simulink model "ScriptDemo"  (R2022b)
settings: configuration reference "TmVcThermal_Configuration_sub" (kept outside this file)
undefined symbols (not defined in the file or in its folder): aaaa, bbbb, cTmComprCtrl_D_u8HvacFlowTable_db, cTmComprCtrl_D_u8HvacFlowTable_sw, cTmComprCtrl_n_i16ChillCmpIMax, cTmComprCtrl_n_i16ChillCmpIMin, cTmComprCtrl_n_i16ChillCmpIMin666, cTmComprCtrl_n_i16ChillCmpPMax, cTmComprCtrl_n_i16ChillCmpPMin, cTmComprCtrl_n_i16CmpChillCoolRpmKiMax, cTmComprCtrl_n_i16CmpChillCoolRpmKiMin, cTmComprCtrl_n_i16CmpChillCoolRpmKpMax, cTmComprCtrl_n_i16CmpChillCoolRpmKpMin, cTmComprCtrl_n_i16CmpCoolRpmKiMax, cTmComprCtrl_n_i16CmpCoolRpmKiMin, cTmComprCtrl_n_i16CmpCoolRpmKpMax, cTmComprCtrl_n_i16CmpCoolRpmKpMin, cTmComprCtrl_n_i16SM4CmpHeatKiMax, cTmComprCtrl_n_i16SM4CmpHeatKiMin, cTmComprCtrl_n_i16SM4CmpHeatKpMax, cTmComprCtrl_n_i16SM4CmpHeatKpMin, cTmComprCtrl_n_i16SM5CmpHeatKiMax, cTmComprCtrl_n_i16SM5CmpHeatKiMin, cTmComprCtrl_n_i16SM5CmpHeatKpMax, cTmComprCtrl_n_i16SM5CmpHeatKpMin, cTmComprCtrl_n_i16SM6CmpHeatKiMax, cTmComprCtrl_n_i16SM6CmpHeatKiMin, cTmComprCtrl_n_i16SM6CmpHeatKpMax, cTmComprCtrl_n_i16SM6CmpHeatKpMin, cTmComprCtrl_n_u16CmpMaxSpdFanFltLimt, cTmComprCtrl_n_u16CmpMaxSpdLoSidePFltLimt, cTmComprCtrl_n_u16CmpMaxSpdSensorFltLimt, cTmComprCtrl_n_u16CompMinRpm, cTmComprCtrl_n_u16CompRpmIncThres, cTmComprCtrl_t_u16BattCooltFFPeriod, cTmComprCtrl_t_u16BattCooltPIPeriod, cTmComprCtrl_t_u16CmpCoolFFPeriod, cTmComprCtrl_t_u16CmpCoolPIPeriod, cTmComprCtrl_t_u16CoolCmpChillFFPeriod, cTmComprCtrl_t_u16CoolCmpChillPIPeriod, cTmComprCtrl_t_u16SM4CmpHeatFFPeriod, cTmComprCtrl_t_u16SM4CmpHeatPIPeriod, cTmComprCtrl_t_u16SM5CmpHeatFFPeriod, cTmComprCtrl_t_u16SM5CmpHeatPIPeriod, cTmComprCtrl_t_u16SM6CmpHeatFFPeriod, cTmComprCtrl_t_u16SM6CmpHeatPIPeriod, cTmComprCtrl_Te_EvapClearInteg, cTmComprCtrl_Te_i16HpReqTempSaturoffset, cTmComprCtrl_Te_i16SatLpReplaceDiff, cTmComprCtrl_Te_i16SM3BatDiffStartEvapDecOffset, cTmComprCtrl_Te_i16SM3EvapLo, cTmComprCtrl_Te_i16SM3TBatDiffEntEvapDecOffset, cTmComprCtrl_Te_i16SM3TBatDiffEntEvapDecOffsetQuit, cTmComprCtrl_Te_s32ErrCmpChillPIContinueCoolH, cTmComprCtrl_Te_s32ErrCmpChillPIContinueCoolL, cTmComprCtrl_Te_s32ErrCmpPIContinueChillH, cTmComprCtrl_Te_s32ErrCmpPIContinueChillL, cTmComprCtrl_Te_s32ErrCmpPIContinueCoolH, cTmComprCtrl_Te_s32ErrCmpPIContinueCoolL, cTmComprCtrl_Te_s32ErrCmpPIContinueHeatH ... (+398)
libraries: simulink x846, PCMULib x711, simulink_need_slupdate x4
(part 13 of 49)

== system ScriptDemo/Find/findModBkSpecific/Before ==
  note: % 目的: 为输出端口创建debug 及对应的输入模块
      | [cnt] = createDebug(gcs)
  sTmRefriVlvCtrl_X_s32CEXVPosReqIn : Inport  OutDataTypeStr=single
  sTmRefriVlvCtrl_X_s32EEXVPosReqIn : Inport  Port=2  OutDataTypeStr=single
  sTmRefriVlvCtrl_X_s32BEXVPosReqIn : Inport  Port=3  OutDataTypeStr=single
  yTmRefriVlvCtrl_B_HpcCexvMovEnableIn : Inport  Port=4  OutDataTypeStr=boolean
  sTmRefriVlvCtrl_Z_u8CEXVInitStateIn : Inport  Port=5  OutDataTypeStr=uint8
  yTmRefriVlvCtrl_B_CexvCalibReqIn : Inport  Port=6  OutDataTypeStr=boolean
  yTmRefriVlvCtrl_B_HpcEexvMovEnableIn : Inport  Port=7  OutDataTypeStr=boolean
  sTmRefriVlvCtrl_Z_u8EEXVInitStateIn : Inport  Port=8  OutDataTypeStr=uint8
  yTmRefriVlvCtrl_B_EexvCalibReqIn : Inport  Port=9  OutDataTypeStr=boolean
  yTmRefriVlvCtrl_B_HpcBexvMovEnableIn : Inport  Port=10  OutDataTypeStr=boolean
  sTmRefriVlvCtrl_Z_u8BEXVInitStateIn : Inport  Port=11  OutDataTypeStr=uint8
  yTmRefriVlvCtrl_B_BexvCalibReqIn : Inport  Port=12  OutDataTypeStr=boolean
  sTmRefriVlvCtrl_X_s32SM3BexvMaxPosIn : Inport  Port=13  OutDataTypeStr=single
  yTmRefriVlvCtrl_B_EvapBattTLimBexvEnaIn : Inport  Port=14  OutDataTypeStr=boolean
  sTmRefriVlvCtrl_D_u8EexvRefriSwitchStIn : Inport  Port=15  OutDataTypeStr=uint8
  sTmRefriVlvCtrl_D_u8CexvRefriSwitchStIn : Inport  Port=16  OutDataTypeStr=uint8
  sTmRefriVlvCtrl_D_u8BexvRefriSwitchStIn : Inport  Port=17  OutDataTypeStr=uint8
  OutDebug : PCMULib/Interface/OutdebugRvs  SWI=cTmRefriVlvCtrl_X_s32CEXVPosReq_sw  DBI=cTmRefriVlvCtrl_X_s32CEXVPosReq_db
      settings: SourceProductName=PCMULib
  OutDebug1 : PCMULib/Interface/OutdebugRvs  SWI=cTmRefriVlvCtrl_X_s32EEXVPosReq_sw  DBI=cTmRefriVlvCtrl_X_s32EEXVPosReq_db
      settings: SourceProductName=PCMULib
  OutDebug10 : PCMULib/Interface/OutdebugRvs  SWI=cTmRefriVlvCtrl_Z_u8BEXVInitState_sw  DBI=cTmRefriVlvCtrl_Z_u8BEXVInitState_db
      settings: SourceProductName=PCMULib
  OutDebug11 : PCMULib/Interface/OutdebugRvs  SWI=cTmRefriVlvCtrl_B_BexvCalibReq_sw  DBI=cTmRefriVlvCtrl_B_BexvCalibReq_db
      settings: SourceProductName=PCMULib
  OutDebug12 : PCMULib/Interface/OutdebugRvs  SWI=cTmRefriVlvCtrl_X_s32SM3BexvMaxPos_sw  DBI=cTmRefriVlvCtrl_X_s32SM3BexvMaxPos_db
      settings: SourceProductName=PCMULib
  OutDebug13 : PCMULib/Interface/OutdebugRvs  SWI=cTmRefriVlvCtrl_B_EvapBattTLimBexvEna_sw  DBI=cTmRefriVlvCtrl_B_EvapBattTLimBexvEna_db
      settings: SourceProductName=PCMULib
  OutDebug14 : PCMULib/Interface/OutdebugRvs  SWI=cTmRefriVlvCtrl_D_u8EexvRefriSwitchSt_sw  DBI=cTmRefriVlvCtrl_D_u8EexvRefriSwitchSt_db
      settings: SourceProductName=PCMULib
  OutDebug15 : PCMULib/Interface/OutdebugRvs  SWI=cTmRefriVlvCtrl_D_u8CexvRefriSwitchSt_sw  DBI=cTmRefriVlvCtrl_D_u8CexvRefriSwitchSt_db
      settings: SourceProductName=PCMULib
  OutDebug16 : PCMULib/Interface/OutdebugRvs  SWI=cTmRefriVlvCtrl_D_u8BexvRefriSwitchSt_sw  DBI=cTmRefriVlvCtrl_D_u8BexvRefriSwitchSt_db
      settings: SourceProductName=PCMULib
  OutDebug2 : PCMULib/Interface/OutdebugRvs  SWI=cTmRefriVlvCtrl_X_s32BEXVPosReq_sw  DBI=cTmRefriVlvCtrl_X_s32BEXVPosReq_db
      settings: SourceProductName=PCMULib
  OutDebug3 : PCMULib/Interface/OutdebugRvs  SWI=cTmRefriVlvCtrl_B_HpcCexvMovEnable_sw  DBI=cTmRefriVlvCtrl_B_HpcCexvMovEnable_db
      settings: SourceProductName=PCMULib
  OutDebug4 : PCMULib/Interface/OutdebugRvs  SWI=cTmRefriVlvCtrl_Z_u8CEXVInitState_sw  DBI=cTmRefriVlvCtrl_Z_u8CEXVInitState_db
      settings: SourceProductName=PCMULib
  OutDebug5 : PCMULib/Interface/OutdebugRvs  SWI=cTmRefriVlvCtrl_B_CexvCalibReq_sw  DBI=cTmRefriVlvCtrl_B_CexvCalibReq_db
      settings: SourceProductName=PCMULib
  OutDebug6 : PCMULib/Interface/OutdebugRvs  SWI=cTmRefriVlvCtrl_B_HpcEexvMovEnable_sw  DBI=cTmRefriVlvCtrl_B_HpcEexvMovEnable_db
      settings: SourceProductName=PCMULib
  OutDebug7 : PCMULib/Interface/OutdebugRvs  SWI=cTmRefriVlvCtrl_Z_u8EEXVInitState_sw  DBI=cTmRefriVlvCtrl_Z_u8EEXVInitState_db
      settings: SourceProductName=PCMULib
  OutDebug8 : PCMULib/Interface/OutdebugRvs  SWI=cTmRefriVlvCtrl_B_EexvCalibReq_sw  DBI=cTmRefriVlvCtrl_B_EexvCalibReq_db
      settings: SourceProductName=PCMULib
  OutDebug9 : PCMULib/Interface/OutdebugRvs  SWI=cTmRefriVlvCtrl_B_HpcBexvMovEnable_sw  DBI=cTmRefriVlvCtrl_B_HpcBexvMovEnable_db
      settings: SourceProductName=PCMULib
  sTmRefriVlvCtrl_X_s32CEXVPosReq : Outport  OutDataTypeStr=single
  sTmRefriVlvCtrl_X_s32EEXVPosReq : Outport  Port=2  OutDataTypeStr=single
  sTmRefriVlvCtrl_X_s32BEXVPosReq : Outport  Port=3  OutDataTypeStr=single
  yTmRefriVlvCtrl_B_HpcCexvMovEnable : Outport  Port=4  OutDataTypeStr=boolean
  sTmRefriVlvCtrl_Z_u8CEXVInitState : Outport  Port=5  OutDataTypeStr=uint8
  yTmRefriVlvCtrl_B_CexvCalibReq : Outport  Port=6  OutDataTypeStr=boolean
  yTmRefriVlvCtrl_B_HpcEexvMovEnable : Outport  Port=7  OutDataTypeStr=boolean
  sTmRefriVlvCtrl_Z_u8EEXVInitState : Outport  Port=8  OutDataTypeStr=uint8
  yTmRefriVlvCtrl_B_EexvCalibReq : Outport  Port=9  OutDataTypeStr=boolean
  yTmRefriVlvCtrl_B_HpcBexvMovEnable : Outport  Port=10  OutDataTypeStr=boolean
  sTmRefriVlvCtrl_Z_u8BEXVInitState : Outport  Port=11  OutDataTypeStr=uint8
  yTmRefriVlvCtrl_B_BexvCalibReq : Outport  Port=12  OutDataTypeStr=boolean
  sTmRefriVlvCtrl_X_s32SM3BexvMaxPos : Outport  Port=13  OutDataTypeStr=single
  yTmRefriVlvCtrl_B_EvapBattTLimBexvEna : Outport  Port=14  OutDataTypeStr=boolean
  sTmRefriVlvCtrl_D_u8EexvRefriSwitchSt : Outport  Port=15  OutDataTypeStr=uint8
  sTmRefriVlvCtrl_D_u8CexvRefriSwitchSt : Outport  Port=16  OutDataTypeStr=uint8
  sTmRefriVlvCtrl_D_u8BexvRefriSwitchSt : Outport  Port=17  OutDataTypeStr=uint8
  wires:
  sTmRefriVlvCtrl_X_s32SM3BexvMaxPosIn/1 -> OutDebug12/1
  OutDebug12/1 -> sTmRefriVlvCtrl_X_s32SM3BexvMaxPos/1
  sTmRefriVlvCtrl_X_s32BEXVPosReqIn/1 -> OutDebug2/1
  OutDebug2/1 -> sTmRefriVlvCtrl_X_s32BEXVPosReq/1
  OutDebug16/1 -> sTmRefriVlvCtrl_D_u8BexvRefriSwitchSt/1
  sTmRefriVlvCtrl_D_u8EexvRefriSwitchStIn/1 -> OutDebug14/1
  OutDebug5/1 -> yTmRefriVlvCtrl_B_CexvCalibReq/1
  OutDebug3/1 -> yTmRefriVlvCtrl_B_HpcCexvMovEnable/1
  sTmRefriVlvCtrl_Z_u8CEXVInitStateIn/1 -> OutDebug4/1
  OutDebug4/1 -> sTmRefriVlvCtrl_Z_u8CEXVInitState/1
  sTmRefriVlvCtrl_D_u8BexvRefriSwitchStIn/1 -> OutDebug16/1
  OutDebug1/1 -> sTmRefriVlvCtrl_X_s32EEXVPosReq/1
  OutDebug14/1 -> sTmRefriVlvCtrl_D_u8EexvRefriSwitchSt/1
  yTmRefriVlvCtrl_B_CexvCalibReqIn/1 -> OutDebug5/1
  sTmRefriVlvCtrl_X_s32EEXVPosReqIn/1 -> OutDebug1/1
  yTmRefriVlvCtrl_B_HpcCexvMovEnableIn/1 -> OutDebug3/1
  yTmRefriVlvCtrl_B_EvapBattTLimBexvEnaIn/1 -> OutDebug13/1
  OutDebug13/1 -> yTmRefriVlvCtrl_B_EvapBattTLimBexvEna/1
  sTmRefriVlvCtrl_Z_u8BEXVInitStateIn/1 -> OutDebug10/1
  OutDebug10/1 -> sTmRefriVlvCtrl_Z_u8BEXVInitState/1
  sTmRefriVlvCtrl_D_u8CexvRefriSwitchStIn/1 -> OutDebug15/1
  OutDebug15/1 -> sTmRefriVlvCtrl_D_u8CexvRefriSwitchSt/1
  OutDebug/1 -> sTmRefriVlvCtrl_X_s32CEXVPosReq/1
  OutDebug7/1 -> sTmRefriVlvCtrl_Z_u8EEXVInitState/1
  OutDebug8/1 -> yTmRefriVlvCtrl_B_EexvCalibReq/1
  yTmRefriVlvCtrl_B_EexvCalibReqIn/1 -> OutDebug8/1
  sTmRefriVlvCtrl_X_s32CEXVPosReqIn/1 -> OutDebug/1
  OutDebug6/1 -> yTmRefriVlvCtrl_B_HpcEexvMovEnable/1
  yTmRefriVlvCtrl_B_HpcEexvMovEnableIn/1 -> OutDebug6/1
  sTmRefriVlvCtrl_Z_u8EEXVInitStateIn/1 -> OutDebug7/1
  yTmRefriVlvCtrl_B_HpcBexvMovEnableIn/1 -> OutDebug9/1
  OutDebug9/1 -> yTmRefriVlvCtrl_B_HpcBexvMovEnable/1
  yTmRefriVlvCtrl_B_BexvCalibReqIn/1 -> OutDebug11/1
  OutDebug11/1 -> yTmRefriVlvCtrl_B_BexvCalibReq/1

== system ScriptDemo/Find/findNameMdOut/SM1 ==
  In : Inport
  rSM1_D_u32AccmKp : Outport
  wires:
  In/1 -> rSM1_D_u32AccmKp/1

== system ScriptDemo/Find/findNameMdOut/SM2 ==
  In : Inport
  rSM2_D_u32AccmKp : Outport
  wires:
  In/1 -> rSM2_D_u32AccmKp/1

== system ScriptDemo/Find/findNameMdOut/SM3 ==
  In : Inport
  sTmComprCtrl_D_u32AccmKpSM3 : Outport
  wires:
  In/1 -> sTmComprCtrl_D_u32AccmKpSM3/1

== system ScriptDemo/Find/findNameMdOut/SM4 ==
  In : Inport
  sTmComprCtrl_D_u32AccmKpSM4 : Outport
  wires:
  In/1 -> sTmComprCtrl_D_u32AccmKpSM4/1

== system ScriptDemo/WorkFlow/Step1_CreateSoftwareReq/Fun666666_Req26245_DemoSub1 ==
  note: 压缩机不满足开启条件
  note: 压缩机允许功率
  note: 压缩机满足开启条件
  note: <模型信息: Fun666666_Req26245_DemoSub1>
      |
      | 【输入端口】
      | sTmIn_Pw_s32HvCoolgAllwd
      | xTmComprCtrl_B_CompOnReqCompOn
      |
      | 【输出端口】
      | sTmComprCtrl_Pw_s32ElacCmprMaxState
      | yTmComprCtrl_B_HpcCoolgLimd
      |
      | 【标定量】
      | cTmComprCtrl_n_i16ChillCmpIMin
      |
      | 创建时间: 2025-03-13 10:25:04
  sTmIn_Pw_s32HvCoolgAllwd : Inport  OutDataTypeStr=single
  xTmComprCtrl_B_CompOnReqCompOn : Inport  Port=2  OutDataTypeStr=boolean
  Compare To Constant : simulink/Logic and Bit Operations/Compare To Constant  relop=>=  const=6500  OutDataTypeStr=boolean
  Compare To Constant1 : simulink/Logic and Bit Operations/Compare To Constant  relop===  const=6500  OutDataTypeStr=boolean
  Constant1 : Constant  Commented=on  Value=cTmComprCtrl_n_i16ChillCmpIMin666  OutDataTypeStr=single
  Constant2 : Constant  Value=cTmComprCtrl_n_i16ChillCmpIMin  OutDataTypeStr=single
  Constant4 : Constant  Value=6500  OutDataTypeStr=single
  Relay : Relay  Commented=on  OnSwitchValue=aaaa  OffSwitchValue=bbbb
  Switch1 : Switch  Criteria=u2 ~= 0  SaturateOnIntegerOverflow=off  InputSameDT=off
  Switch3 : Switch  Criteria=u2 ~= 0  Threshold=6500  SaturateOnIntegerOverflow=off  InputSameDT=off
  sTmComprCtrl_Pw_s32ElacCmprMaxState : Outport  OutDataTypeStr=single
  yTmComprCtrl_B_HpcCoolgLimd : Outport  Port=2  OutDataTypeStr=boolean
  wires:
  Compare To Constant1/1 -> [yTmComprCtrl_B_HpcCoolgLimd]
  Switch1/1 -> [sTmComprCtrl_Pw_s32ElacCmprMaxState], Compare To Constant1/1
  Constant2/1 -> Switch1/3
  Constant4/1 -> Switch3/1
  Compare To Constant/1 -> Switch3/2
  Switch3/1 -> Switch1/1
  [xTmComprCtrl_B_CompOnReqCompOn] -> Switch1/2
  [sTmIn_Pw_s32HvCoolgAllwd] -> Switch3/3, Compare To Constant/1
  sTmIn_Pw_s32HvCoolgAllwd/1 -> [sTmIn_Pw_s32HvCoolgAllwd]
  xTmComprCtrl_B_CompOnReqCompOn/1 -> [xTmComprCtrl_B_CompOnReqCompOn]
  [sTmComprCtrl_Pw_s32ElacCmprMaxState] -> sTmComprCtrl_Pw_s32ElacCmprMaxState/1
  [yTmComprCtrl_B_HpcCoolgLimd] -> yTmComprCtrl_B_HpcCoolgLimd/1

== system ScriptDemo/WorkFlow/Step1_CreateSoftwareReq/Fun666666_Req26246_DemoSub2 ==

== system ScriptDemo/WorkFlow/Step1_CreateSoftwareReq/Fun666666_Req26247_DemoSub3 ==

== system ScriptDemo/WorkFlow/Step1_CreateSoftwareReq/Fun666666_Req26248_DemoSub4 ==

== system ScriptDemo/WorkFlow/Step1_CreateSoftwareReq/Fun666666_Req26249_DemoSub5 ==

== system ScriptDemo/WorkFlow/Step1_CreateSoftwareReq/Fun888888_Req26250_DemoSub6 ==

== system ScriptDemo/WorkFlow/Step1_CreateSoftwareReq/Fun888888_Req26251_DemoSub7 ==

== system ScriptDemo/WorkFlow/Step1_CreateSoftwareReq/Fun888888_Req26252_DemoSub8 ==

== system ScriptDemo/WorkFlow/Step1_CreateSoftwareReq/Fun888888_Req26253_DemoSub9 ==

== system ScriptDemo/WorkFlow/Step1_CreateSoftwareReq/Fun888888_Req26254_DemoSub10 ==

== system ScriptDemo/WorkFlow/Step1_CreateSubModel/Fun666666_Req26245_DemoSub1 ==

== system ScriptDemo/WorkFlow/Step1_CreateSubModel/Fun666666_Req26246_DemoSub2 ==

== system ScriptDemo/WorkFlow/Step1_CreateSubModel/Fun666666_Req26247_DemoSub3 ==

== system ScriptDemo/WorkFlow/Step1_CreateSubModel/Fun666666_Req26248_DemoSub4 ==

== system ScriptDemo/WorkFlow/Step1_CreateSubModel/Fun666666_Req26249_DemoSub5 ==

== system ScriptDemo/WorkFlow/Step1_CreateSubModel/Fun888888_Req26250_DemoSub6 ==

== system ScriptDemo/WorkFlow/Step1_CreateSubModel/Fun888888_Req26251_DemoSub7 ==

== system ScriptDemo/WorkFlow/Step1_CreateSubModel/Fun888888_Req26252_DemoSub8 ==

== system ScriptDemo/WorkFlow/Step1_CreateSubModel/Fun888888_Req26253_DemoSub9 ==

== system ScriptDemo/WorkFlow/Step1_CreateSubModel/Fun888888_Req26254_DemoSub10 ==

== system ScriptDemo/createHarness/ID31659_OffCodeState/bk ==
  note: 第1位
  note: 输出: 0
  note: 输出: 4
  note: 第5位
  note: 第24位
  note: 第5、6、10、13、25、26位
  note: 第8位
  note: 输出: 1
  note: 输出: 5
  note: 输出: 3
  note: 输出: 2
  note: 第3、4、7、15、16、17、18、19、20、21、22、23、27、28、29、30
  note: 输出: 6
  note: 输出: 7
  sTmComprCtrl_D_u32AcOffCode : Inport  OutDataTypeStr=uint32
  sTmRefriModeMgr_D_u8HPCurMode : Inport  Port=2
  Bitwise Operator : simulink/Logic and Bit Operations/Bitwise Operator  logicop=AND  UseBitMask=on  BitMask=0x00000001  BitMaskRealWorld=Stored Integer
  Bitwise Operator2 : simulink/Logic and Bit Operations/Bitwise Operator  logicop=AND  UseBitMask=on  BitMask=0x01000000  BitMaskRealWorld=Stored Integer
  Bitwise Operator3 : simulink/Logic and Bit Operations/Bitwise Operator  logicop=AND  UseBitMask=on  BitMask=0x00000100  BitMaskRealWorld=Stored Integer
  Bitwise Operator4 : simulink/Logic and Bit Operations/Bitwise Operator  logicop=AND  UseBitMask=on  BitMask=0x20  BitMaskRealWorld=Stored Integer
  Bitwise Operator5 : simulink/Logic and Bit Operations/Bitwise Operator  logicop=AND  UseBitMask=on  BitMask=0x78FF804C  BitMaskRealWorld=Stored Integer
  Bitwise Operator6 : simulink/Logic and Bit Operations/Bitwise Operator  logicop=AND  UseBitMask=on  BitMask=0x06002460  BitMaskRealWorld=Stored Integer
  Compare To Constant{,1..7} (8 alike) : simulink/Logic and Bit Operations/Compare To Constant  relop=>  const=0  OutDataTypeStr=uint8
  Constant : Constant  Value=0  OutDataTypeStr=uint64
  Constant1 : Constant  Value=[1 21 3 23]  OutDataTypeStr=uint64
  Constant2 : Constant  Value=[2 22 4 5 6 7]  OutDataTypeStr=uint64
  Logical Operator : Logic  AllPortsSameDT=off  OutDataTypeStr=boolean
  Logical Operator1 : Logic  Operator=OR  Inputs=1  AllPortsSameDT=off  OutDataTypeStr=boolean
  Logical Operator2 : Logic  Operator=OR  Inputs=1  AllPortsSameDT=off  OutDataTypeStr=boolean
  Logical Operator3 : Logic  AllPortsSameDT=off  OutDataTypeStr=boolean
  Merge : Merge  Inputs=8
  Relational Operator : RelationalOperator  Operator===  OutDataTypeStr=boolean  RndMeth=Simplest  InputSameDT=off
  Relational Operator1 : RelationalOperator  Operator===  OutDataTypeStr=boolean  RndMeth=Simplest  InputSameDT=off
  Relational Operator2 : RelationalOperator  Operator===  OutDataTypeStr=boolean  RndMeth=Simplest  InputSameDT=off
  Subsystem : Subsystem
  Subsystem1 : Subsystem
  Subsystem2 : Subsystem
  Subsystem3 : Subsystem
  Subsystem4 : Subsystem
  Subsystem5 : Subsystem
  Subsystem6 : Subsystem
  Subsystem7 : Subsystem
  sTmComprCtrl_D_u8AirCondCmpsrStats : Outport  OutDataTypeStr=uint8
  wires:
  Compare To Constant2/1 -> Subsystem2/Enable
  sTmComprCtrl_D_u32AcOffCode/1 -> Relational Operator/1, Bitwise Operator6/1, Bitwise Operator5/1, Bitwise Operator4/1, Bitwise Operator3/1, Bitwise Operator2/1, Bitwise Operator/1
  Subsystem5/1(sTmComprCtrl_D_u8AirCondCmpsrStats) -> Merge/6
  Compare To Constant6/1 -> Subsystem6/Enable
  Constant2/1 -> Relational Operator2/2
  Subsystem7/1(sTmComprCtrl_D_u8AirCondCmpsrStats) -> Merge/8
  Logical Operator3/1 -> Compare To Constant7/1
  Subsystem/1(sTmComprCtrl_D_u8AirCondCmpsrStats) -> Merge/1
  Relational Operator/1 -> Logical Operator3/1, Logical Operator/1
  Compare To Constant4/1 -> Subsystem4/Enable
  Merge/1 -> sTmComprCtrl_D_u8AirCondCmpsrStats/1
  Constant1/1 -> Relational Operator1/2
  Bitwise Operator2/1 -> Compare To Constant1/1
  Subsystem6/1(sTmComprCtrl_D_u8AirCondCmpsrStats) -> Merge/7
  Subsystem2/1(sTmComprCtrl_D_u8AirCondCmpsrStats) -> Merge/3
  Subsystem1/1(sTmComprCtrl_D_u8AirCondCmpsrStats) -> Merge/2
  Bitwise Operator6/1 -> Compare To Constant5/1
  Relational Operator1/1 -> Logical Operator1/1
  Subsystem4/1(sTmComprCtrl_D_u8AirCondCmpsrStats) -> Merge/5
  Bitwise Operator5/1 -> Compare To Constant4/1
  Subsystem3/1(sTmComprCtrl_D_u8AirCondCmpsrStats) -> Merge/4
  Relational Operator2/1 -> Logical Operator2/1
  Logical Operator/1 -> Compare To Constant6/1
  Bitwise Operator/1 -> Compare To Constant/1
  Compare To Constant3/1 -> Subsystem3/Enable
  Bitwise Operator3/1 -> Compare To Constant2/1
  sTmRefriModeMgr_D_u8HPCurMode/1 -> Relational Operator2/1, Relational Operator1/1
  Compare To Constant/1 -> Subsystem/Enable
  Bitwise Operator4/1 -> Compare To Constant3/1
  Logical Operator1/1 -> Logical Operator/2
  Compare To Constant7/1 -> Subsystem7/Enable
  Compare To Constant1/1 -> Subsystem1/Enable
  Constant/1 -> Relational Operator/2
  Logical Operator2/1 -> Logical Operator3/2
  Compare To Constant5/1 -> Subsystem5/Enable

== system ScriptDemo/Change/changeModSize/After/Subsystem ==
  sTmSigProces_Te_s32EvapFanReqRamp : Inport  OutDataTypeStr=single
  sTmDiag_D_u8TeEvapFltSt : Inport  Port=2  OutDataTypeStr=uint8
  sTmIn_D_u8HeatPump : Inport  Port=3  OutDataTypeStr=uint8
  sTmIn_X_s32ClimtRcirc : Inport  Port=4  OutDataTypeStr=single
  sTmComprCtrl_D_u8HvacFlowLevel : Inport  Port=5  OutDataTypeStr=uint8
  sTmSigProces_Te_s32EvapFanFilter : Inport  Port=6  OutDataTypeStr=single
  sTmSigProces_Te_s32SatLp : Inport  Port=7  OutDataTypeStr=single
  xTmComprCtrl_B_CompOnReqCompOn : Inport  Port=8  OutDataTypeStr=boolean
  yTmRefriModeMgr_B_CoolOCRMode : Inport  Port=9  OutDataTypeStr=boolean
  sTmSigProces_Pw_i16ReqPwrForCool : Inport  Port=10  OutDataTypeStr=int16
  rSM2SM22_n_u16DisOverrideValue : Outport  OutDataTypeStr=uint16
  rSM2SM22_t_u16PIPeriod : Outport  Port=2  OutDataTypeStr=uint16
  rSM2SM22_Te_s32UpErrStop : Outport  Port=3  OutDataTypeStr=single
  rSM2SM22_n_u16ComprRpmFF : Outport  Port=4  OutDataTypeStr=uint16
  rSM2SM22_n_u16ComprRpmKp : Outport  Port=5  OutDataTypeStr=uint16
  rSM2SM22_n_u16ComprRpmKi : Outport  Port=6  OutDataTypeStr=uint16
  rSM2SM22_Te_s32LowErrStop : Outport  Port=7  OutDataTypeStr=single
  rSM2SM22_n_i16KpUpLimit : Outport  Port=8  OutDataTypeStr=int16
  rSM2SM22_n_i16KpLowLimit : Outport  Port=9  OutDataTypeStr=int16
  rSM2SM22_n_i16KiUpLimit : Outport  Port=10  OutDataTypeStr=int16
  rSM2SM22_n_i16KiLowLimit : Outport  Port=11  OutDataTypeStr=int16
  rSM2SM22_B_Enable : Outport  Port=12  OutDataTypeStr=boolean
  rSM2SM22_Te_s32TempError : Outport  Port=13  OutDataTypeStr=single
  wires:
  sTmSigProces_Te_s32SatLp/1 -> [sTmSigProces_Te_s32SatLp]
  [rTmComprCtrl_n_u16ComprRpmKp] -> rSM2SM22_n_u16ComprRpmKp/1
  sTmDiag_D_u8TeEvapFltSt/1 -> [sTmDiag_D_u8TeEvapFltSt]
  sTmIn_X_s32ClimtRcirc/1 -> [sTmIn_X_s32ClimtRcirc]
  sTmSigProces_Te_s32EvapFanReqRamp/1 -> [sTmSigProces_Te_s32EvapFanReqRamp]
  sTmIn_D_u8HeatPump/1 -> [sTmIn_D_u8HeatPump]
  sTmSigProces_Te_s32EvapFanFilter/1 -> [sTmSigProces_Te_s32EvapFanFilter]
  [rTmComprCtrl_n_u16ComprRpmFF] -> rSM2SM22_n_u16ComprRpmFF/1
  xTmComprCtrl_B_CompOnReqCompOn/1 -> [xTmComprCtrl_B_CompOnReqCompOn]
  [rTmComprCtrl_Te_s32UpErrStop] -> rSM2SM22_Te_s32UpErrStop/1
  [rTmComprCtrl_t_u16PIPeriod] -> rSM2SM22_t_u16PIPeriod/1
  ? -> [yTmRefriModeMgr_B_CoolModeInCycle]
  sTmComprCtrl_D_u8HvacFlowLevel/1 -> [sTmComprCtrl_D_u8HvacFlowLevel]
  ? -> [sTmSigProces_Te_s32TAmb]
  [rTmComprCtrl_Te_s32TempError] -> rSM2SM22_Te_s32TempError/1
  [rTmComprCtrl_n_i16KiUpLimit] -> rSM2SM22_n_i16KiUpLimit/1
  [rTmComprCtrl_Te_s32LowErrStop] -> rSM2SM22_Te_s32LowErrStop/1
  [rTmComprCtrl_n_i16KiLowLimit] -> rSM2SM22_n_i16KiLowLimit/1
  [rTmComprCtrl_n_i16KpLowLimit] -> rSM2SM22_n_i16KpLowLimit/1
  yTmRefriModeMgr_B_CoolOCRMode/1 -> [yTmRefriModeMgr_B_CoolOCRMode]
  [rTmComprCtrl_n_i16KpUpLimit] -> rSM2SM22_n_i16KpUpLimit/1
  sTmSigProces_Pw_i16ReqPwrForCool/1 -> [sTmSigProces_Pw_i16ReqPwrForCool]
  [xTmComprCtrl_B_Enable] -> rSM2SM22_B_Enable/1
  [rTmComprCtrl_n_u16DisOverrideValue] -> rSM2SM22_n_u16DisOverrideValue/1
  [rTmComprCtrl_n_u16ComprRpmKi] -> rSM2SM22_n_u16ComprRpmKi/1

== system ScriptDemo/Change/changeModSizeGcs/Before/Subsystem ==
  rTmComprCtrl_n_u16CompRpmReqModeOut : Inport  OutDataTypeStr=uint16
  sTmDiag_D_u8CmprDischrgTFltSt : Inport  Port=2  OutDataTypeStr=uint8
  sTmDiag_D_u8FanFltSt : Inport  Port=3  OutDataTypeStr=uint8
  sTmDiag_D_u8HiSidePFltSt : Inport  Port=4  OutDataTypeStr=uint8
  sTmDiag_D_u8OutrCondOutTFltSt : Inport  Port=5  OutDataTypeStr=uint8
  sTmIn_n_s32ElacCmprActl : Inport  Port=6  OutDataTypeStr=single
  sTmIn_v_s32VehSpdLgt : Inport  Port=7  OutDataTypeStr=single
  sTmRefriModeMgr_D_u8HpFmCmd : Inport  Port=8  OutDataTypeStr=uint8
  sTmSigProces_Pw_i16ReqPwrForHeat : Inport  Port=9  OutDataTypeStr=int16
  sTmSigProces_Te_s32CompDischarge : Inport  Port=10  OutDataTypeStr=single
  sTmSigProces_md_u16BlwCool : Inport  Port=11  OutDataTypeStr=uint16
  sTmSigProces_p_u16PHighSide : Inport  Port=12  OutDataTypeStr=uint16
  sTmSigProces_p_u16PLowSide : Inport  Port=13  OutDataTypeStr=uint16
  sTmIn_D_u8HeatPump : Inport  Port=14  OutDataTypeStr=uint8
  sTmIn_D_u8ElecDriveline : Inport  Port=15
  sTmSigProces_md_u16BlwHeat : Inport  Port=16  OutDataTypeStr=uint16
  sTmDiag_D_u8LoSidePFltSt : Inport  Port=17  OutDataTypeStr=uint8
  xTmComprCtrl_B_CompOnReqCompOn : Inport  Port=18  OutDataTypeStr=boolean
  rTmComprCtrl_n_u16CompRpmReqFilter : Outport  OutDataTypeStr=uint16
  xTmComprCtrl_B_KeepRpm : Outport  Port=2  OutDataTypeStr=boolean
  xFilter_B_ComprStop : Outport  Port=3  OutDataTypeStr=boolean
  sFilter_n_u16CompMaxRpm : Outport  Port=4  OutDataTypeStr=uint16
  rFilter_p_u16AcHiSideHiCut : Outport  Port=5  OutDataTypeStr=uint16
  rFilter_p_u16CmpLimitNormalP : Outport  Port=6  OutDataTypeStr=uint16
  rFilter_p_u16CmpLimitLowP : Outport  Port=7  OutDataTypeStr=uint16
  rFilter_p_u16CmpLimitMidP : Outport  Port=8  OutDataTypeStr=uint16
  rFilter_p_u16CmpLimitShutDownP : Outport  Port=9  OutDataTypeStr=uint16
  xTmComprCtrl_B_ReduceRpm : Outport  Port=10  OutDataTypeStr=boolean
  wires:
  ? -> [sTmRefriModeMgr_D_u8HPCurMode]
  sTmIn_n_s32ElacCmprActl/1 -> [sTmIn_n_s32ElacCmprActl]
  [rTmComprCtrl_p_u16AcHiSideHiCut] -> rFilter_p_u16AcHiSideHiCut/1
  sTmIn_D_u8HeatPump/1 -> [sTmIn_D_u8HeatPump]
  sTmSigProces_md_u16BlwCool/1 -> [sTmSigProces_md_u16BlwCool]
  sTmDiag_D_u8OutrCondOutTFltSt/1 -> [sTmDiag_D_u8OutrCondOutTFltSt]
  ? -> [sTmSigProces_Te_s32TAmb]
  sTmSigProces_md_u16BlwHeat/1 -> [sTmSigProces_md_u16BlwHeat]
  [rTmComprCtrl_p_u16CmpLimitShutDownP] -> rFilter_p_u16CmpLimitShutDownP/1
  sTmRefriModeMgr_D_u8HpFmCmd/1 -> [sTmRefriModeMgr_D_u8HpFmCmd]
  [rTmComprCtrl_p_u16CmpLimitLowP] -> rFilter_p_u16CmpLimitLowP/1
  sTmDiag_D_u8LoSidePFltSt/1 -> [sTmDiag_D_u8LoSidePFltSt]
  sTmSigProces_p_u16PLowSide/1 -> [sTmSigProces_p_u16PLowSide]
  [rTmComprCtrl_n_u16CompRpmReqCompOn] -> rTmComprCtrl_n_u16CompRpmReqFilter/1
  [xTmComprCtrl_B_ComprStop] -> xFilter_B_ComprStop/1
  sTmIn_D_u8ElecDriveline/1 -> [sTmIn_D_u8ElecDriveline]
  sTmDiag_D_u8HiSidePFltSt/1 -> [sTmDiag_D_u8HiSidePFltSt]
  [sTmComprCtrl_n_u16CompMaxRpm] -> sFilter_n_u16CompMaxRpm/1
  ? -> [sTmSigProces_D_u8CarChrgMode]
  [xTmComprCtrl_B_KeepRpm] -> xTmComprCtrl_B_KeepRpm/1
  sTmDiag_D_u8CmprDischrgTFltSt/1 -> [sTmDiag_D_u8CmprDischrgTFltSt]
  sTmSigProces_p_u16PHighSide/1 -> [sTmSigProces_p_u16PHighSide]
  xTmComprCtrl_B_CompOnReqCompOn/1 -> [xTmComprCtrl_B_CompOnReqCompOn]
  sTmSigProces_Te_s32CompDischarge/1 -> [sTmSigProces_Te_s32CompDischarge]
  [rTmComprCtrl_p_u16CmpLimitMidP] -> rFilter_p_u16CmpLimitMidP/1
  [rTmComprCtrl_p_u16CmpLimitNormalP] -> rFilter_p_u16CmpLimitNormalP/1
  sTmIn_v_s32VehSpdLgt/1 -> [sTmIn_v_s32VehSpdLgt]
  [xTmComprCtrl_B_ReduceRpm] -> xTmComprCtrl_B_ReduceRpm/1
  sTmSigProces_Pw_i16ReqPwrForHeat/1 -> [sTmSigProces_Pw_i16ReqPwrForHeat]
  sTmDiag_D_u8FanFltSt/1 -> [sTmDiag_D_u8FanFltSt]
  rTmComprCtrl_n_u16CompRpmReqModeOut/1 -> [rTmComprCtrl_n_u16CompRpmReqModeOut]

== system ScriptDemo/Change/changeModSizeGcs/Before/Subsystem1 ==
  rTmComprCtrl_n_u16CompRpmReqModeOut : Inport  OutDataTypeStr=uint16
  sTmDiag_D_u8CmprDischrgTFltSt : Inport  Port=2  OutDataTypeStr=uint8
  sTmDiag_D_u8FanFltSt : Inport  Port=3  OutDataTypeStr=uint8
  sTmDiag_D_u8HiSidePFltSt : Inport  Port=4  OutDataTypeStr=uint8
  sTmDiag_D_u8OutrCondOutTFltSt : Inport  Port=5  OutDataTypeStr=uint8
  sTmIn_n_s32ElacCmprActl : Inport  Port=6  OutDataTypeStr=single
  sTmIn_v_s32VehSpdLgt : Inport  Port=7  OutDataTypeStr=single
  sTmRefriModeMgr_D_u8HpFmCmd : Inport  Port=8  OutDataTypeStr=uint8
  sTmSigProces_Pw_i16ReqPwrForHeat : Inport  Port=9  OutDataTypeStr=int16
  sTmSigProces_Te_s32CompDischarge : Inport  Port=10  OutDataTypeStr=single
  rTmComprCtrl_n_u16CompRpmReqFilter : Outport  OutDataTypeStr=uint16
  xTmComprCtrl_B_KeepRpm : Outport  Port=2  OutDataTypeStr=boolean
  xFilter_B_ComprStop : Outport  Port=3  OutDataTypeStr=boolean
  sFilter_n_u16CompMaxRpm : Outport  Port=4  OutDataTypeStr=uint16
  rFilter_p_u16AcHiSideHiCut : Outport  Port=5  OutDataTypeStr=uint16
  rFilter_p_u16CmpLimitNormalP : Outport  Port=6  OutDataTypeStr=uint16
  rFilter_p_u16CmpLimitLowP : Outport  Port=7  OutDataTypeStr=uint16
  rFilter_p_u16CmpLimitMidP : Outport  Port=8  OutDataTypeStr=uint16
  rFilter_p_u16CmpLimitShutDownP : Outport  Port=9  OutDataTypeStr=uint16
  xTmComprCtrl_B_ReduceRpm : Outport  Port=10  OutDataTypeStr=boolean
  wires:
  ? -> [sTmRefriModeMgr_D_u8HPCurMode]
  sTmIn_n_s32ElacCmprActl/1 -> [sTmIn_n_s32ElacCmprActl]
  [rTmComprCtrl_p_u16AcHiSideHiCut] -> rFilter_p_u16AcHiSideHiCut/1
  sTmDiag_D_u8OutrCondOutTFltSt/1 -> [sTmDiag_D_u8OutrCondOutTFltSt]
  ? -> [sTmSigProces_Te_s32TAmb]
  [rTmComprCtrl_p_u16CmpLimitShutDownP] -> rFilter_p_u16CmpLimitShutDownP/1
  sTmRefriModeMgr_D_u8HpFmCmd/1 -> [sTmRefriModeMgr_D_u8HpFmCmd]
  [rTmComprCtrl_p_u16CmpLimitLowP] -> rFilter_p_u16CmpLimitLowP/1
  [rTmComprCtrl_n_u16CompRpmReqCompOn] -> rTmComprCtrl_n_u16CompRpmReqFilter/1
  [xTmComprCtrl_B_ComprStop] -> xFilter_B_ComprStop/1
  sTmDiag_D_u8HiSidePFltSt/1 -> [sTmDiag_D_u8HiSidePFltSt]
  [sTmComprCtrl_n_u16CompMaxRpm] -> sFilter_n_u16CompMaxRpm/1
  [xTmComprCtrl_B_KeepRpm] -> xTmComprCtrl_B_KeepRpm/1
  sTmDiag_D_u8CmprDischrgTFltSt/1 -> [sTmDiag_D_u8CmprDischrgTFltSt]
  sTmSigProces_Te_s32CompDischarge/1 -> [sTmSigProces_Te_s32CompDischarge]
  [rTmComprCtrl_p_u16CmpLimitMidP] -> rFilter_p_u16CmpLimitMidP/1
  [rTmComprCtrl_p_u16CmpLimitNormalP] -> rFilter_p_u16CmpLimitNormalP/1
  sTmIn_v_s32VehSpdLgt/1 -> [sTmIn_v_s32VehSpdLgt]
  [xTmComprCtrl_B_ReduceRpm] -> xTmComprCtrl_B_ReduceRpm/1
  sTmSigProces_Pw_i16ReqPwrForHeat/1 -> [sTmSigProces_Pw_i16ReqPwrForHeat]
  sTmDiag_D_u8FanFltSt/1 -> [sTmDiag_D_u8FanFltSt]
  rTmComprCtrl_n_u16CompRpmReqModeOut/1 -> [rTmComprCtrl_n_u16CompRpmReqModeOut]

== system ScriptDemo/Change/changeModSizeGcs/Before/Subsystem2 ==
  rTmComprCtrl_n_u16CompRpmReqModeOut : Inport  OutDataTypeStr=uint16
  sTmDiag_D_u8CmprDischrgTFltSt : Inport  Port=2  OutDataTypeStr=uint8
  sTmDiag_D_u8FanFltSt : Inport  Port=3  OutDataTypeStr=uint8
  sTmDiag_D_u8HiSidePFltSt : Inport  Port=4  OutDataTypeStr=uint8
  sTmDiag_D_u8OutrCondOutTFltSt : Inport  Port=5  OutDataTypeStr=uint8
  sTmIn_n_s32ElacCmprActl : Inport  Port=6  OutDataTypeStr=single
  sTmIn_v_s32VehSpdLgt : Inport  Port=7  OutDataTypeStr=single
  sTmRefriModeMgr_D_u8HpFmCmd : Inport  Port=8  OutDataTypeStr=uint8
  sTmSigProces_Pw_i16ReqPwrForHeat : Inport  Port=9  OutDataTypeStr=int16
  sTmSigProces_Te_s32CompDischarge : Inport  Port=10  OutDataTypeStr=single
  sTmSigProces_md_u16BlwCool : Inport  Port=11  OutDataTypeStr=uint16
  sTmSigProces_p_u16PHighSide : Inport  Port=12  OutDataTypeStr=uint16
  sTmSigProces_p_u16PLowSide : Inport  Port=13  OutDataTypeStr=uint16
  sTmIn_D_u8HeatPump : Inport  Port=14  OutDataTypeStr=uint8
  sTmIn_D_u8ElecDriveline : Inport  Port=15
  sTmSigProces_md_u16BlwHeat : Inport  Port=16  OutDataTypeStr=uint16
  sTmDiag_D_u8LoSidePFltSt : Inport  Port=17  OutDataTypeStr=uint8
  xTmComprCtrl_B_CompOnReqCompOn : Inport  Port=18  OutDataTypeStr=boolean
  rTmComprCtrl_n_u16CompRpmReqFilter : Outport  OutDataTypeStr=uint16
  xTmComprCtrl_B_KeepRpm : Outport  Port=2  OutDataTypeStr=boolean
  xFilter_B_ComprStop : Outport  Port=3  OutDataTypeStr=boolean
  sFilter_n_u16CompMaxRpm : Outport  Port=4  OutDataTypeStr=uint16
  rFilter_p_u16AcHiSideHiCut : Outport  Port=5  OutDataTypeStr=uint16
  rFilter_p_u16CmpLimitNormalP : Outport  Port=6  OutDataTypeStr=uint16
  rFilter_p_u16CmpLimitLowP : Outport  Port=7  OutDataTypeStr=uint16
  rFilter_p_u16CmpLimitMidP : Outport  Port=8  OutDataTypeStr=uint16
  rFilter_p_u16CmpLimitShutDownP : Outport  Port=9  OutDataTypeStr=uint16
  xTmComprCtrl_B_ReduceRpm : Outport  Port=10  OutDataTypeStr=boolean
  wires:
  ? -> [sTmRefriModeMgr_D_u8HPCurMode]
  sTmIn_n_s32ElacCmprActl/1 -> [sTmIn_n_s32ElacCmprActl]
  [rTmComprCtrl_p_u16AcHiSideHiCut] -> rFilter_p_u16AcHiSideHiCut/1
  sTmIn_D_u8HeatPump/1 -> [sTmIn_D_u8HeatPump]
  sTmSigProces_md_u16BlwCool/1 -> [sTmSigProces_md_u16BlwCool]
  sTmDiag_D_u8OutrCondOutTFltSt/1 -> [sTmDiag_D_u8OutrCondOutTFltSt]
  ? -> [sTmSigProces_Te_s32TAmb]
  sTmSigProces_md_u16BlwHeat/1 -> [sTmSigProces_md_u16BlwHeat]
  [rTmComprCtrl_p_u16CmpLimitShutDownP] -> rFilter_p_u16CmpLimitShutDownP/1
  sTmRefriModeMgr_D_u8HpFmCmd/1 -> [sTmRefriModeMgr_D_u8HpFmCmd]
  [rTmComprCtrl_p_u16CmpLimitLowP] -> rFilter_p_u16CmpLimitLowP/1
  sTmDiag_D_u8LoSidePFltSt/1 -> [sTmDiag_D_u8LoSidePFltSt]
  sTmSigProces_p_u16PLowSide/1 -> [sTmSigProces_p_u16PLowSide]
  [rTmComprCtrl_n_u16CompRpmReqCompOn] -> rTmComprCtrl_n_u16CompRpmReqFilter/1
  [xTmComprCtrl_B_ComprStop] -> xFilter_B_ComprStop/1
  sTmIn_D_u8ElecDriveline/1 -> [sTmIn_D_u8ElecDriveline]
  sTmDiag_D_u8HiSidePFltSt/1 -> [sTmDiag_D_u8HiSidePFltSt]
  [sTmComprCtrl_n_u16CompMaxRpm] -> sFilter_n_u16CompMaxRpm/1
  ? -> [sTmSigProces_D_u8CarChrgMode]
  [xTmComprCtrl_B_KeepRpm] -> xTmComprCtrl_B_KeepRpm/1
  sTmDiag_D_u8CmprDischrgTFltSt/1 -> [sTmDiag_D_u8CmprDischrgTFltSt]
  sTmSigProces_p_u16PHighSide/1 -> [sTmSigProces_p_u16PHighSide]
  xTmComprCtrl_B_CompOnReqCompOn/1 -> [xTmComprCtrl_B_CompOnReqCompOn]
  sTmSigProces_Te_s32CompDischarge/1 -> [sTmSigProces_Te_s32CompDischarge]
  [rTmComprCtrl_p_u16CmpLimitMidP] -> rFilter_p_u16CmpLimitMidP/1
  [rTmComprCtrl_p_u16CmpLimitNormalP] -> rFilter_p_u16CmpLimitNormalP/1
  sTmIn_v_s32VehSpdLgt/1 -> [sTmIn_v_s32VehSpdLgt]
  [xTmComprCtrl_B_ReduceRpm] -> xTmComprCtrl_B_ReduceRpm/1
  sTmSigProces_Pw_i16ReqPwrForHeat/1 -> [sTmSigProces_Pw_i16ReqPwrForHeat]
  sTmDiag_D_u8FanFltSt/1 -> [sTmDiag_D_u8FanFltSt]
  rTmComprCtrl_n_u16CompRpmReqModeOut/1 -> [rTmComprCtrl_n_u16CompRpmReqModeOut]

== system ScriptDemo/Change/changeModSizeGcs/Before/Subsystem3 ==
  rTmComprCtrl_n_u16CompRpmReqModeOut : Inport  OutDataTypeStr=uint16
  sTmDiag_D_u8CmprDischrgTFltSt : Inport  Port=2  OutDataTypeStr=uint8
  sTmDiag_D_u8FanFltSt : Inport  Port=3  OutDataTypeStr=uint8
  sTmDiag_D_u8HiSidePFltSt : Inport  Port=4  OutDataTypeStr=uint8
  sTmDiag_D_u8OutrCondOutTFltSt : Inport  Port=5  OutDataTypeStr=uint8
  sTmIn_n_s32ElacCmprActl : Inport  Port=6  OutDataTypeStr=single
  sTmIn_v_s32VehSpdLgt : Inport  Port=7  OutDataTypeStr=single
  sTmRefriModeMgr_D_u8HpFmCmd : Inport  Port=8  OutDataTypeStr=uint8
  sTmSigProces_Pw_i16ReqPwrForHeat : Inport  Port=9  OutDataTypeStr=int16
  sTmSigProces_Te_s32CompDischarge : Inport  Port=10  OutDataTypeStr=single
  sTmSigProces_md_u16BlwCool : Inport  Port=11  OutDataTypeStr=uint16
  sTmSigProces_p_u16PHighSide : Inport  Port=12  OutDataTypeStr=uint16
  sTmSigProces_p_u16PLowSide : Inport  Port=13  OutDataTypeStr=uint16
  sTmIn_D_u8HeatPump : Inport  Port=14  OutDataTypeStr=uint8
  sTmIn_D_u8ElecDriveline : Inport  Port=15
  sTmSigProces_md_u16BlwHeat : Inport  Port=16  OutDataTypeStr=uint16
  sTmDiag_D_u8LoSidePFltSt : Inport  Port=17  OutDataTypeStr=uint8
  xTmComprCtrl_B_CompOnReqCompOn : Inport  Port=18  OutDataTypeStr=boolean
  rTmComprCtrl_n_u16CompRpmReqFilter : Outport  OutDataTypeStr=uint16
  xTmComprCtrl_B_KeepRpm : Outport  Port=2  OutDataTypeStr=boolean
  xFilter_B_ComprStop : Outport  Port=3  OutDataTypeStr=boolean
  sFilter_n_u16CompMaxRpm : Outport  Port=4  OutDataTypeStr=uint16
  rFilter_p_u16AcHiSideHiCut : Outport  Port=5  OutDataTypeStr=uint16
  rFilter_p_u16CmpLimitNormalP : Outport  Port=6  OutDataTypeStr=uint16
  rFilter_p_u16CmpLimitLowP : Outport  Port=7  OutDataTypeStr=uint16
  rFilter_p_u16CmpLimitMidP : Outport  Port=8  OutDataTypeStr=uint16
  rFilter_p_u16CmpLimitShutDownP : Outport  Port=9  OutDataTypeStr=uint16
  xTmComprCtrl_B_ReduceRpm : Outport  Port=10  OutDataTypeStr=boolean
  wires:
  ? -> [sTmRefriModeMgr_D_u8HPCurMode]
  sTmIn_n_s32ElacCmprActl/1 -> [sTmIn_n_s32ElacCmprActl]
  [rTmComprCtrl_p_u16AcHiSideHiCut] -> rFilter_p_u16AcHiSideHiCut/1
  sTmIn_D_u8HeatPump/1 -> [sTmIn_D_u8HeatPump]
  sTmSigProces_md_u16BlwCool/1 -> [sTmSigProces_md_u16BlwCool]
  sTmDiag_D_u8OutrCondOutTFltSt/1 -> [sTmDiag_D_u8OutrCondOutTFltSt]
  ? -> [sTmSigProces_Te_s32TAmb]
  sTmSigProces_md_u16BlwHeat/1 -> [sTmSigProces_md_u16BlwHeat]
  [rTmComprCtrl_p_u16CmpLimitShutDownP] -> rFilter_p_u16CmpLimitShutDownP/1
  sTmRefriModeMgr_D_u8HpFmCmd/1 -> [sTmRefriModeMgr_D_u8HpFmCmd]
  [rTmComprCtrl_p_u16CmpLimitLowP] -> rFilter_p_u16CmpLimitLowP/1
  sTmDiag_D_u8LoSidePFltSt/1 -> [sTmDiag_D_u8LoSidePFltSt]
  sTmSigProces_p_u16PLowSide/1 -> [sTmSigProces_p_u16PLowSide]
  [rTmComprCtrl_n_u16CompRpmReqCompOn] -> rTmComprCtrl_n_u16CompRpmReqFilter/1
  [xTmComprCtrl_B_ComprStop] -> xFilter_B_ComprStop/1
  sTmIn_D_u8ElecDriveline/1 -> [sTmIn_D_u8ElecDriveline]
  sTmDiag_D_u8HiSidePFltSt/1 -> [sTmDiag_D_u8HiSidePFltSt]
  [sTmComprCtrl_n_u16CompMaxRpm] -> sFilter_n_u16CompMaxRpm/1
  ? -> [sTmSigProces_D_u8CarChrgMode]
  [xTmComprCtrl_B_KeepRpm] -> xTmComprCtrl_B_KeepRpm/1
  sTmDiag_D_u8CmprDischrgTFltSt/1 -> [sTmDiag_D_u8CmprDischrgTFltSt]
  sTmSigProces_p_u16PHighSide/1 -> [sTmSigProces_p_u16PHighSide]
  xTmComprCtrl_B_CompOnReqCompOn/1 -> [xTmComprCtrl_B_CompOnReqCompOn]
  sTmSigProces_Te_s32CompDischarge/1 -> [sTmSigProces_Te_s32CompDischarge]
  [rTmComprCtrl_p_u16CmpLimitMidP] -> rFilter_p_u16CmpLimitMidP/1
  [rTmComprCtrl_p_u16CmpLimitNormalP] -> rFilter_p_u16CmpLimitNormalP/1
  sTmIn_v_s32VehSpdLgt/1 -> [sTmIn_v_s32VehSpdLgt]
  [xTmComprCtrl_B_ReduceRpm] -> xTmComprCtrl_B_ReduceRpm/1
  sTmSigProces_Pw_i16ReqPwrForHeat/1 -> [sTmSigProces_Pw_i16ReqPwrForHeat]
  sTmDiag_D_u8FanFltSt/1 -> [sTmDiag_D_u8FanFltSt]
  rTmComprCtrl_n_u16CompRpmReqModeOut/1 -> [rTmComprCtrl_n_u16CompRpmReqModeOut]

== system ScriptDemo/Change/changeModSizeGcs/Before1/Subsystem ==
  rTmComprCtrl_n_u16CompRpmReqModeOut : Inport  OutDataTypeStr=uint16
  sTmDiag_D_u8CmprDischrgTFltSt : Inport  Port=2  OutDataTypeStr=uint8
  sTmDiag_D_u8FanFltSt : Inport  Port=3  OutDataTypeStr=uint8
  sTmDiag_D_u8HiSidePFltSt : Inport  Port=4  OutDataTypeStr=uint8
  sTmDiag_D_u8OutrCondOutTFltSt : Inport  Port=5  OutDataTypeStr=uint8
  sTmIn_n_s32ElacCmprActl : Inport  Port=6  OutDataTypeStr=single
  sTmIn_v_s32VehSpdLgt : Inport  Port=7  OutDataTypeStr=single
  sTmRefriModeMgr_D_u8HpFmCmd : Inport  Port=8  OutDataTypeStr=uint8
  sTmSigProces_Pw_i16ReqPwrForHeat : Inport  Port=9  OutDataTypeStr=int16
  sTmSigProces_Te_s32CompDischarge : Inport  Port=10  OutDataTypeStr=single
  sTmSigProces_md_u16BlwCool : Inport  Port=11  OutDataTypeStr=uint16
  sTmSigProces_p_u16PHighSide : Inport  Port=12  OutDataTypeStr=uint16
  sTmSigProces_p_u16PLowSide : Inport  Port=13  OutDataTypeStr=uint16
  sTmIn_D_u8HeatPump : Inport  Port=14  OutDataTypeStr=uint8
  sTmIn_D_u8ElecDriveline : Inport  Port=15
  sTmSigProces_md_u16BlwHeat : Inport  Port=16  OutDataTypeStr=uint16
  sTmDiag_D_u8LoSidePFltSt : Inport  Port=17  OutDataTypeStr=uint8
  xTmComprCtrl_B_CompOnReqCompOn : Inport  Port=18  OutDataTypeStr=boolean
  rTmComprCtrl_n_u16CompRpmReqFilter : Outport  OutDataTypeStr=uint16
  xTmComprCtrl_B_KeepRpm : Outport  Port=2  OutDataTypeStr=boolean
  xFilter_B_ComprStop : Outport  Port=3  OutDataTypeStr=boolean
  sFilter_n_u16CompMaxRpm : Outport  Port=4  OutDataTypeStr=uint16
  rFilter_p_u16AcHiSideHiCut : Outport  Port=5  OutDataTypeStr=uint16
  rFilter_p_u16CmpLimitNormalP : Outport  Port=6  OutDataTypeStr=uint16
  rFilter_p_u16CmpLimitLowP : Outport  Port=7  OutDataTypeStr=uint16
  rFilter_p_u16CmpLimitMidP : Outport  Port=8  OutDataTypeStr=uint16
  rFilter_p_u16CmpLimitShutDownP : Outport  Port=9  OutDataTypeStr=uint16
  xTmComprCtrl_B_ReduceRpm : Outport  Port=10  OutDataTypeStr=boolean
  wires:
  ? -> [sTmRefriModeMgr_D_u8HPCurMode]
  sTmIn_n_s32ElacCmprActl/1 -> [sTmIn_n_s32ElacCmprActl]
  [rTmComprCtrl_p_u16AcHiSideHiCut] -> rFilter_p_u16AcHiSideHiCut/1
  sTmIn_D_u8HeatPump/1 -> [sTmIn_D_u8HeatPump]
  sTmSigProces_md_u16BlwCool/1 -> [sTmSigProces_md_u16BlwCool]
  sTmDiag_D_u8OutrCondOutTFltSt/1 -> [sTmDiag_D_u8OutrCondOutTFltSt]
  ? -> [sTmSigProces_Te_s32TAmb]
  sTmSigProces_md_u16BlwHeat/1 -> [sTmSigProces_md_u16BlwHeat]
  [rTmComprCtrl_p_u16CmpLimitShutDownP] -> rFilter_p_u16CmpLimitShutDownP/1
  sTmRefriModeMgr_D_u8HpFmCmd/1 -> [sTmRefriModeMgr_D_u8HpFmCmd]
  [rTmComprCtrl_p_u16CmpLimitLowP] -> rFilter_p_u16CmpLimitLowP/1
  sTmDiag_D_u8LoSidePFltSt/1 -> [sTmDiag_D_u8LoSidePFltSt]
  sTmSigProces_p_u16PLowSide/1 -> [sTmSigProces_p_u16PLowSide]
  [rTmComprCtrl_n_u16CompRpmReqCompOn] -> rTmComprCtrl_n_u16CompRpmReqFilter/1
  [xTmComprCtrl_B_ComprStop] -> xFilter_B_ComprStop/1
  sTmIn_D_u8ElecDriveline/1 -> [sTmIn_D_u8ElecDriveline]
  sTmDiag_D_u8HiSidePFltSt/1 -> [sTmDiag_D_u8HiSidePFltSt]
  [sTmComprCtrl_n_u16CompMaxRpm] -> sFilter_n_u16CompMaxRpm/1
  ? -> [sTmSigProces_D_u8CarChrgMode]
  [xTmComprCtrl_B_KeepRpm] -> xTmComprCtrl_B_KeepRpm/1
  sTmDiag_D_u8CmprDischrgTFltSt/1 -> [sTmDiag_D_u8CmprDischrgTFltSt]
  sTmSigProces_p_u16PHighSide/1 -> [sTmSigProces_p_u16PHighSide]
  xTmComprCtrl_B_CompOnReqCompOn/1 -> [xTmComprCtrl_B_CompOnReqCompOn]
  sTmSigProces_Te_s32CompDischarge/1 -> [sTmSigProces_Te_s32CompDischarge]
  [rTmComprCtrl_p_u16CmpLimitMidP] -> rFilter_p_u16CmpLimitMidP/1
  [rTmComprCtrl_p_u16CmpLimitNormalP] -> rFilter_p_u16CmpLimitNormalP/1
  sTmIn_v_s32VehSpdLgt/1 -> [sTmIn_v_s32VehSpdLgt]
  [xTmComprCtrl_B_ReduceRpm] -> xTmComprCtrl_B_ReduceRpm/1
  sTmSigProces_Pw_i16ReqPwrForHeat/1 -> [sTmSigProces_Pw_i16ReqPwrForHeat]
  sTmDiag_D_u8FanFltSt/1 -> [sTmDiag_D_u8FanFltSt]
  rTmComprCtrl_n_u16CompRpmReqModeOut/1 -> [rTmComprCtrl_n_u16CompRpmReqModeOut]

== system ScriptDemo/Change/changeModSizeGcs/Before1/Subsystem1 ==
  rTmComprCtrl_n_u16CompRpmReqModeOut : Inport  OutDataTypeStr=uint16
  sTmDiag_D_u8CmprDischrgTFltSt : Inport  Port=2  OutDataTypeStr=uint8
  sTmDiag_D_u8FanFltSt : Inport  Port=3  OutDataTypeStr=uint8
  sTmDiag_D_u8HiSidePFltSt : Inport  Port=4  OutDataTypeStr=uint8
  sTmDiag_D_u8OutrCondOutTFltSt : Inport  Port=5  OutDataTypeStr=uint8
  sTmIn_n_s32ElacCmprActl : Inport  Port=6  OutDataTypeStr=single
  sTmIn_v_s32VehSpdLgt : Inport  Port=7  OutDataTypeStr=single
  sTmRefriModeMgr_D_u8HpFmCmd : Inport  Port=8  OutDataTypeStr=uint8
  sTmSigProces_Pw_i16ReqPwrForHeat : Inport  Port=9  OutDataTypeStr=int16
  sTmSigProces_Te_s32CompDischarge : Inport  Port=10  OutDataTypeStr=single
  rTmComprCtrl_n_u16CompRpmReqFilter : Outport  OutDataTypeStr=uint16
  xTmComprCtrl_B_KeepRpm : Outport  Port=2  OutDataTypeStr=boolean
  xFilter_B_ComprStop : Outport  Port=3  OutDataTypeStr=boolean
  sFilter_n_u16CompMaxRpm : Outport  Port=4  OutDataTypeStr=uint16
  rFilter_p_u16AcHiSideHiCut : Outport  Port=5  OutDataTypeStr=uint16
  rFilter_p_u16CmpLimitNormalP : Outport  Port=6  OutDataTypeStr=uint16
  rFilter_p_u16CmpLimitLowP : Outport  Port=7  OutDataTypeStr=uint16
  rFilter_p_u16CmpLimitMidP : Outport  Port=8  OutDataTypeStr=uint16
  rFilter_p_u16CmpLimitShutDownP : Outport  Port=9  OutDataTypeStr=uint16
  xTmComprCtrl_B_ReduceRpm : Outport  Port=10  OutDataTypeStr=boolean
  wires:
  ? -> [sTmRefriModeMgr_D_u8HPCurMode]
  sTmIn_n_s32ElacCmprActl/1 -> [sTmIn_n_s32ElacCmprActl]
  [rTmComprCtrl_p_u16AcHiSideHiCut] -> rFilter_p_u16AcHiSideHiCut/1
  sTmDiag_D_u8OutrCondOutTFltSt/1 -> [sTmDiag_D_u8OutrCondOutTFltSt]
  ? -> [sTmSigProces_Te_s32TAmb]
  [rTmComprCtrl_p_u16CmpLimitShutDownP] -> rFilter_p_u16CmpLimitShutDownP/1
  sTmRefriModeMgr_D_u8HpFmCmd/1 -> [sTmRefriModeMgr_D_u8HpFmCmd]
  [rTmComprCtrl_p_u16CmpLimitLowP] -> rFilter_p_u16CmpLimitLowP/1
  [rTmComprCtrl_n_u16CompRpmReqCompOn] -> rTmComprCtrl_n_u16CompRpmReqFilter/1
  [xTmComprCtrl_B_ComprStop] -> xFilter_B_ComprStop/1
  sTmDiag_D_u8HiSidePFltSt/1 -> [sTmDiag_D_u8HiSidePFltSt]
  [sTmComprCtrl_n_u16CompMaxRpm] -> sFilter_n_u16CompMaxRpm/1
  [xTmComprCtrl_B_KeepRpm] -> xTmComprCtrl_B_KeepRpm/1
  sTmDiag_D_u8CmprDischrgTFltSt/1 -> [sTmDiag_D_u8CmprDischrgTFltSt]
  sTmSigProces_Te_s32CompDischarge/1 -> [sTmSigProces_Te_s32CompDischarge]
  [rTmComprCtrl_p_u16CmpLimitMidP] -> rFilter_p_u16CmpLimitMidP/1
  [rTmComprCtrl_p_u16CmpLimitNormalP] -> rFilter_p_u16CmpLimitNormalP/1
  sTmIn_v_s32VehSpdLgt/1 -> [sTmIn_v_s32VehSpdLgt]
  [xTmComprCtrl_B_ReduceRpm] -> xTmComprCtrl_B_ReduceRpm/1
  sTmSigProces_Pw_i16ReqPwrForHeat/1 -> [sTmSigProces_Pw_i16ReqPwrForHeat]
  sTmDiag_D_u8FanFltSt/1 -> [sTmDiag_D_u8FanFltSt]
  rTmComprCtrl_n_u16CompRpmReqModeOut/1 -> [rTmComprCtrl_n_u16CompRpmReqModeOut]

== system ScriptDemo/Change/changeModSizeGcs/Before1/Subsystem2 ==
  rTmComprCtrl_n_u16CompRpmReqModeOut : Inport  OutDataTypeStr=uint16
  sTmDiag_D_u8CmprDischrgTFltSt : Inport  Port=2  OutDataTypeStr=uint8
  sTmDiag_D_u8FanFltSt : Inport  Port=3  OutDataTypeStr=uint8
  sTmDiag_D_u8HiSidePFltSt : Inport  Port=4  OutDataTypeStr=uint8
  sTmDiag_D_u8OutrCondOutTFltSt : Inport  Port=5  OutDataTypeStr=uint8
  sTmIn_n_s32ElacCmprActl : Inport  Port=6  OutDataTypeStr=single
  sTmIn_v_s32VehSpdLgt : Inport  Port=7  OutDataTypeStr=single
  sTmRefriModeMgr_D_u8HpFmCmd : Inport  Port=8  OutDataTypeStr=uint8
  sTmSigProces_Pw_i16ReqPwrForHeat : Inport  Port=9  OutDataTypeStr=int16
  sTmSigProces_Te_s32CompDischarge : Inport  Port=10  OutDataTypeStr=single
  sTmSigProces_md_u16BlwCool : Inport  Port=11  OutDataTypeStr=uint16
  sTmSigProces_p_u16PHighSide : Inport  Port=12  OutDataTypeStr=uint16
  sTmSigProces_p_u16PLowSide : Inport  Port=13  OutDataTypeStr=uint16
  sTmIn_D_u8HeatPump : Inport  Port=14  OutDataTypeStr=uint8
  sTmIn_D_u8ElecDriveline : Inport  Port=15
  sTmSigProces_md_u16BlwHeat : Inport  Port=16  OutDataTypeStr=uint16
  sTmDiag_D_u8LoSidePFltSt : Inport  Port=17  OutDataTypeStr=uint8
  xTmComprCtrl_B_CompOnReqCompOn : Inport  Port=18  OutDataTypeStr=boolean
  rTmComprCtrl_n_u16CompRpmReqFilter : Outport  OutDataTypeStr=uint16
  xTmComprCtrl_B_KeepRpm : Outport  Port=2  OutDataTypeStr=boolean
  xFilter_B_ComprStop : Outport  Port=3  OutDataTypeStr=boolean
  sFilter_n_u16CompMaxRpm : Outport  Port=4  OutDataTypeStr=uint16
  rFilter_p_u16AcHiSideHiCut : Outport  Port=5  OutDataTypeStr=uint16
  rFilter_p_u16CmpLimitNormalP : Outport  Port=6  OutDataTypeStr=uint16
  rFilter_p_u16CmpLimitLowP : Outport  Port=7  OutDataTypeStr=uint16
  rFilter_p_u16CmpLimitMidP : Outport  Port=8  OutDataTypeStr=uint16
  rFilter_p_u16CmpLimitShutDownP : Outport  Port=9  OutDataTypeStr=uint16
  xTmComprCtrl_B_ReduceRpm : Outport  Port=10  OutDataTypeStr=boolean
  wires:
  ? -> [sTmRefriModeMgr_D_u8HPCurMode]
  sTmIn_n_s32ElacCmprActl/1 -> [sTmIn_n_s32ElacCmprActl]
  [rTmComprCtrl_p_u16AcHiSideHiCut] -> rFilter_p_u16AcHiSideHiCut/1
  sTmIn_D_u8HeatPump/1 -> [sTmIn_D_u8HeatPump]
  sTmSigProces_md_u16BlwCool/1 -> [sTmSigProces_md_u16BlwCool]
  sTmDiag_D_u8OutrCondOutTFltSt/1 -> [sTmDiag_D_u8OutrCondOutTFltSt]
  ? -> [sTmSigProces_Te_s32TAmb]
  sTmSigProces_md_u16BlwHeat/1 -> [sTmSigProces_md_u16BlwHeat]
  [rTmComprCtrl_p_u16CmpLimitShutDownP] -> rFilter_p_u16CmpLimitShutDownP/1
  sTmRefriModeMgr_D_u8HpFmCmd/1 -> [sTmRefriModeMgr_D_u8HpFmCmd]
  [rTmComprCtrl_p_u16CmpLimitLowP] -> rFilter_p_u16CmpLimitLowP/1
  sTmDiag_D_u8LoSidePFltSt/1 -> [sTmDiag_D_u8LoSidePFltSt]
  sTmSigProces_p_u16PLowSide/1 -> [sTmSigProces_p_u16PLowSide]
  [rTmComprCtrl_n_u16CompRpmReqCompOn] -> rTmComprCtrl_n_u16CompRpmReqFilter/1
  [xTmComprCtrl_B_ComprStop] -> xFilter_B_ComprStop/1
  sTmIn_D_u8ElecDriveline/1 -> [sTmIn_D_u8ElecDriveline]
  sTmDiag_D_u8HiSidePFltSt/1 -> [sTmDiag_D_u8HiSidePFltSt]
  [sTmComprCtrl_n_u16CompMaxRpm] -> sFilter_n_u16CompMaxRpm/1
  ? -> [sTmSigProces_D_u8CarChrgMode]
  [xTmComprCtrl_B_KeepRpm] -> xTmComprCtrl_B_KeepRpm/1
  sTmDiag_D_u8CmprDischrgTFltSt/1 -> [sTmDiag_D_u8CmprDischrgTFltSt]
  sTmSigProces_p_u16PHighSide/1 -> [sTmSigProces_p_u16PHighSide]
  xTmComprCtrl_B_CompOnReqCompOn/1 -> [xTmComprCtrl_B_CompOnReqCompOn]
  sTmSigProces_Te_s32CompDischarge/1 -> [sTmSigProces_Te_s32CompDischarge]
  [rTmComprCtrl_p_u16CmpLimitMidP] -> rFilter_p_u16CmpLimitMidP/1
  [rTmComprCtrl_p_u16CmpLimitNormalP] -> rFilter_p_u16CmpLimitNormalP/1
  sTmIn_v_s32VehSpdLgt/1 -> [sTmIn_v_s32VehSpdLgt]
  [xTmComprCtrl_B_ReduceRpm] -> xTmComprCtrl_B_ReduceRpm/1
  sTmSigProces_Pw_i16ReqPwrForHeat/1 -> [sTmSigProces_Pw_i16ReqPwrForHeat]
  sTmDiag_D_u8FanFltSt/1 -> [sTmDiag_D_u8FanFltSt]
  rTmComprCtrl_n_u16CompRpmReqModeOut/1 -> [rTmComprCtrl_n_u16CompRpmReqModeOut]
